simulink model "example1"  (Simulink 4.00)
settings: Solver=ode45  StartTime=0.0  StopTime=10.0  MaxStep=0.02  RelTol=1e-3
values from neighbouring files (symbols this model uses):
  A = [0  1; 0  -1]    [params.mat]
  Ae = [-9  1; -41  -1]    [params.mat]
  B = [0 1]    [params.mat]
  C = [2 0]    [params.mat]
  G = [4.5 20.5]    [params.mat]
settings Model: LastModifiedBy=gordon

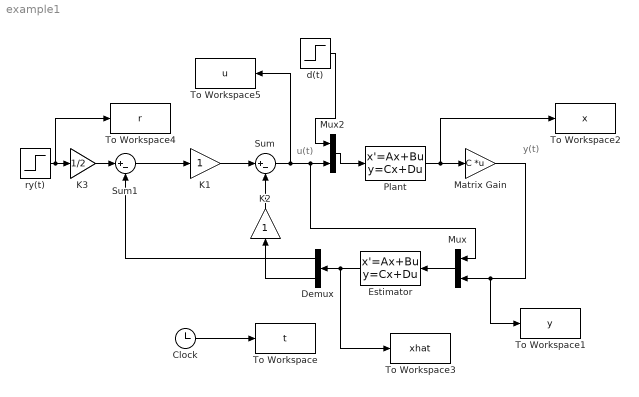
== system example1 ==
  note: u(t)
  note: y(t)
  Clock : Clock
      settings: DisplayTime=off  Decimation=10
  Demux : Demux  Orientation=left  Outputs=2  BusSelectionMode=off
  Estimator : StateSpace  Orientation=left  A=Ae  B=[B G]  C=[1 0;0 1]  D=[0 0;0 0]  X0=0  AbsoluteTolerance=auto  Realization=auto
  K1 : Gain  Gain=1  Multiplication=Element-wise(K.*u)  SaturateOnIntegerOverflow=on
  K2 : Gain  Orientation=up  Gain=1  Multiplication=Element-wise(K.*u)  SaturateOnIntegerOverflow=on
  K3 : Gain  Gain=1/2  Multiplication=Element-wise(K.*u)  SaturateOnIntegerOverflow=on
  Matrix Gain : Gain  Gain=C  Multiplication=Matrix(K*u)  SaturateOnIntegerOverflow=on
  Mux : Mux  Orientation=left  Inputs=2
  Mux2 : Mux  Inputs=2
  Plant : StateSpace  A=A  B=[E B]  C=[1 0;0 1]  D=[0 0; 0 0]  X0=0  AbsoluteTolerance=auto  Realization=auto
  Sum : Sum  Inputs=|+-  SaturateOnIntegerOverflow=on
  Sum1 : Sum  Inputs=|+-  SaturateOnIntegerOverflow=on
  To Workspace : ToWorkspace  VariableName=t  SampleTime=-1  SaveFormat=Array
  To Workspace1 : ToWorkspace  VariableName=y  SampleTime=-1  SaveFormat=Array
  To Workspace2 : ToWorkspace  VariableName=x  SampleTime=-1  SaveFormat=Array
  To Workspace3 : ToWorkspace  VariableName=xhat  SampleTime=-1  SaveFormat=Array
  To Workspace4 : ToWorkspace  VariableName=r  SampleTime=-1  SaveFormat=Array
  To Workspace5 : ToWorkspace  VariableName=u  SampleTime=-1  SaveFormat=Array
  d(t) : Step  Time=1  Before=0  After=0.1  SampleTime=0
  ry(t) : Step  Time=1  Before=0  After=1  SampleTime=0
  wires:
  Mux/1 -> Estimator/1
  Sum/1 -> To Workspace5/1, Mux/1, Mux2/2
  Sum1/1 -> K1/1
  K1/1 -> Sum/1
  K2/1 -> Sum/2
  Demux/2 -> K2/1
  Demux/1 -> Sum1/2
  ry(t)/1 -> K3/1, To Workspace4/1
  K3/1 -> Sum1/1
  Plant/1 -> Matrix Gain/1, To Workspace2/1
  Matrix Gain/1 -> Mux/2, To Workspace1/1
  Clock/1 -> To Workspace/1
  Mux2/1 -> Plant/1
  d(t)/1 -> Mux2/1
  Estimator/1 -> Demux/1, To Workspace3/1
